simulink model "llm_inferencing_control"  (R2025b)
settings: Solver=FixedStepDiscrete  StartTime=0.0  StopTime=30  FixedStep=perturbed.dt  RelTol=1e-3
undefined symbols (not defined in the file): perturbed
settings Model: Creator=hvasudevan  LastModifiedBy=hvasudevan

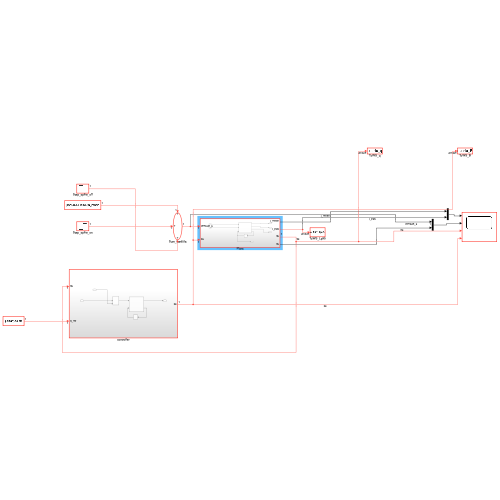
[thumbnail: Simulink's stored preview of the top-level diagram]
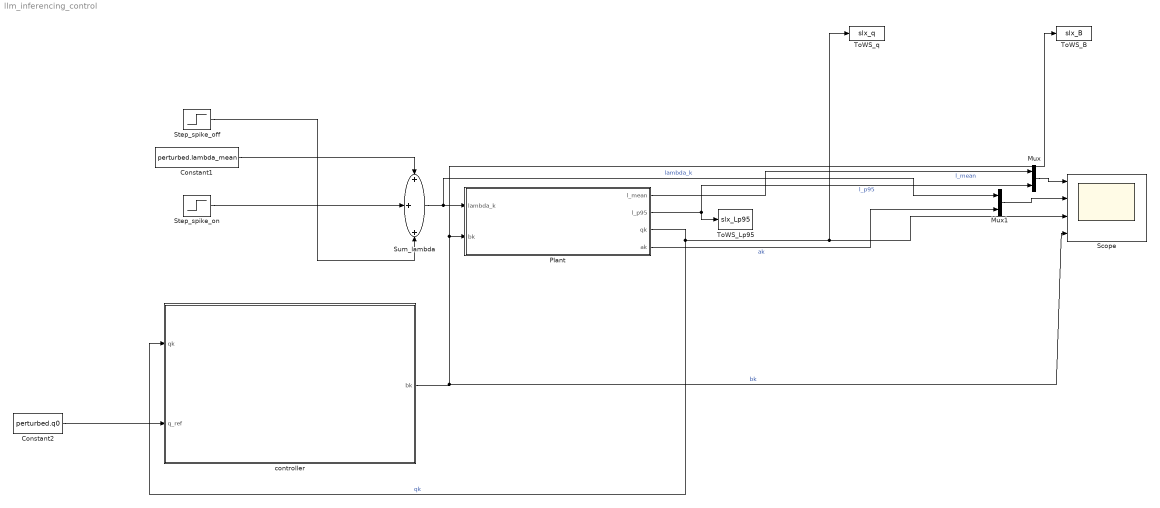
== system llm_inferencing_control ==
  Constant1 : Constant  Value=perturbed.lambda_mean  SampleTime=perturbed.dt
  Constant2 : Constant  Value=perturbed.q0  SampleTime=perturbed.dt
  Mux : Mux  Inputs=2
  Mux1 : Mux  Inputs=2
  Plant : Subsystem
  Scope : Scope  NumInputPorts=4
      settings: ActiveDisplayYMinimum=111.04524983188305  ActiveDisplayYMaximum=461.80657853882258
  Step_spike_off : Step  Time=15  After=-perturbed.lambda_mean  SampleTime=perturbed.dt
  Step_spike_on : Step  Time=5  After=perturbed.lambda_mean  SampleTime=perturbed.dt
  Sum_lambda : Sum  Inputs=+++
  ToWS_B : ToWorkspace  VariableName=slx_B  SampleTime=-1
  ToWS_Lp95 : ToWorkspace  VariableName=slx_Lp95  SampleTime=-1
  ToWS_q : ToWorkspace  VariableName=slx_q  SampleTime=-1
  controller : Subsystem
  wires:
  Step_spike_off/1 -> Sum_lambda/3
  Plant/3(qk) -> controller/1(qk), Scope/3, ToWS_q/1  "qk"
  Plant/2(l_p95) -> Mux/2, ToWS_Lp95/1  "l_p95"
  Plant/1(l_mean) -> Mux/1  "l_mean"
  Step_spike_on/1 -> Sum_lambda/2
  Constant1/1 -> Sum_lambda/1
  Sum_lambda/1 -> Mux1/1, Plant/1(lambda_k)  "lambda_k"
  controller/1(bk) -> ToWS_B/1, Plant/2(bk), Scope/4  "bk"
  Constant2/1 -> controller/2(q_ref)
  Mux/1 -> Scope/1
  Mux1/1 -> Scope/2
  Plant/4(ak) -> Mux1/2  "ak"

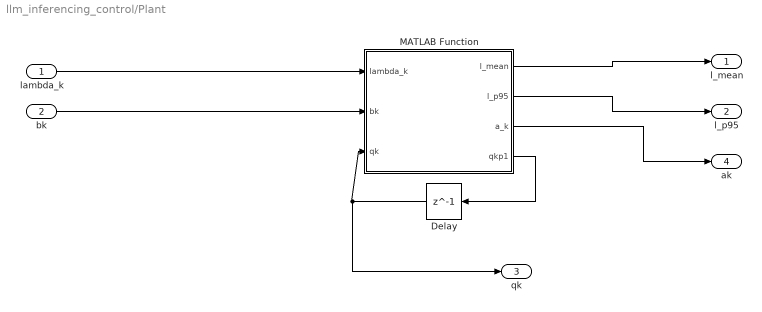
== system llm_inferencing_control/Plant ==
  lambda_k : Inport
  bk : Inport  Port=2
  Delay : Delay  DelayLength=1  InitialCondition=perturbed.q0  InputProcessing=Columns as channels (frame based)
  MATLAB Function : MATLAB Function  TreatAsAtomicUnit=on
  l_mean : Outport
  l_p95 : Outport  Port=2
  qk : Outport  Port=3
  ak : Outport  Port=4
  wires:
  MATLAB Function/2(l_p95) -> l_p95/1
  Delay/1 -> qk/1, MATLAB Function/3(qk)
  bk/1 -> MATLAB Function/2(bk)
  MATLAB Function/4(qkp1) -> Delay/1
  lambda_k/1 -> MATLAB Function/1(lambda_k)
  MATLAB Function/1(l_mean) -> l_mean/1
  MATLAB Function/3(a_k) -> ak/1

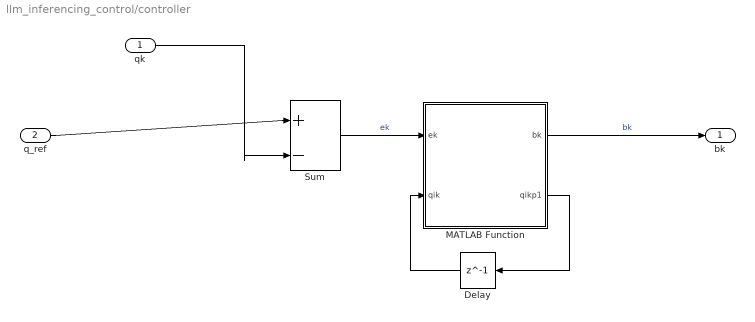
== system llm_inferencing_control/controller ==
  qk : Inport
  q_ref : Inport  Port=2
  Delay : Delay  DelayLength=1  InitialCondition=0  InputProcessing=Columns as channels (frame based)
  MATLAB Function : MATLAB Function  TreatAsAtomicUnit=on
  Sum : Sum  Inputs=|+-
  bk : Outport
  wires:
  MATLAB Function/1(bk) -> bk/1  "bk"
  MATLAB Function/2(qikp1) -> Delay/1
  Sum/1 -> MATLAB Function/1(ek)  "ek"
  qk/1 -> Sum/2
  Delay/1 -> MATLAB Function/2(qik)
  q_ref/1 -> Sum/1

== matlab function llm_inferencing_control/controller/MATLAB Function ==
  data: ek input; qik input; bk output; controller parameter; qikp1 output
function [bk, qikp1] = controller(ek, qik, controller)

q_max = controller.q_max;
B0    = controller.B0;
K_q   = controller.K_aug(1);
K_i   = controller.K_aug(2);
k_aug   = controller.K_aug;

% Saturate error and integrator state to [-q_max, q_max]
% ek can be negative (queue above setpoint) so bounds are symmetric
ek_sat  = min(max(ek,  -q_max), q_max);
qik_sat = min(max(qik, -q_max), q_max);

% Integrator update (Franklin 8.5.1: xi[k+1] = xi[k] + e[k])
qikp1 = qik_sat + ek_sat;
ek_vec = [ek_sat;qik_sat];

% Control law: dB = K_q*ek - K_i*qik  (since ek=-Dq, law is -K_q*Dq - K_i*xi)
% Full batch size: B = B0 + dB
bk = B0 + k_aug * ek_vec;

== matlab function llm_inferencing_control/Plant/MATLAB Function ==
  data: lambda_k input; bk input; l_mean output; qk input; l_p95 output; a_k output; qkp1 output; perturbed parameter
function [l_mean, l_p95, a_k, qkp1] = fcn(lambda_k, bk, qk, perturbed)
%% STATISTICAL PLANT - Chapter 2
%% Replaces deterministic arrivals and closed-form p95 with:
%%   - True Poisson arrivals: a[k] ~ Poisson(lambda_k)
%%   - Per-tick latency sample with additive noise
%%   - Empirical rolling p95 over a 60-sample window
%%
%% Everything else (queue equation, latency formula, parameters)
%% is identical to Chapter 1.

persistent L_buf buf_idx buf_full
N = 60;
if isempty(L_buf)
    %% Warm-start buffer at target so outer loop sees zero error at t=0.
    %% Without this the cold buffer reads L_p95~0 and winds the integrator.
    L_buf    = perturbed.L_p95_target * ones(1, N);
    buf_idx  = 0;
    buf_full = true;
end

alpha = perturbed.alpha;
gam   = perturbed.gamma;
beta  = perturbed.beta;
delta = perturbed.delta;

%% True Poisson arrivals (not Gaussian approx — avoids fat-tail spikes)
a_k = poissrnd(max(0, lambda_k));

%% Queue state equation — identical to Chapter 1
qkp1 = max(0, qk + a_k - bk);

%% Latency sample this tick
bk_safe = max(1, bk);
l_det   = alpha*bk + gam*bk^2 + beta*qk;
l_samp  = l_det + (delta / sqrt(bk_safe)) * randn();

%% Update circular buffer
buf_idx = mod(buf_idx, N) + 1;
L_buf(buf_idx) = l_samp;

%% Rolling statistics
if buf_full
    data = L_buf;
else
    data = L_buf(1 : buf_idx);
end

l_mean = mean(data);
sorted = sort(data);
idx95  = max(1, ceil(0.95 * length(sorted)));
l_p95  = sorted(idx95);

end
